simulink model "P2319ASW01"  (R2022b)
settings: configuration reference "SharedConfig" (kept outside this file)
libraries: simulink x3
settings Model: DataDictionary=P2319ASW01.sldd  Creator=Kevin  LastModifiedBy=Max Kolesnikov
settings ConfigSetRef: SourceName=SharedConfig

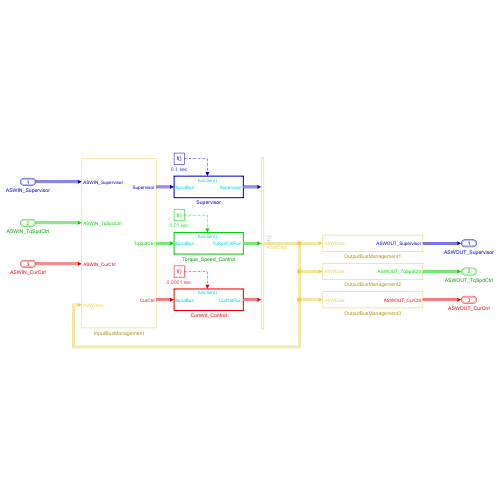
[thumbnail: Simulink's stored preview of the top-level diagram]
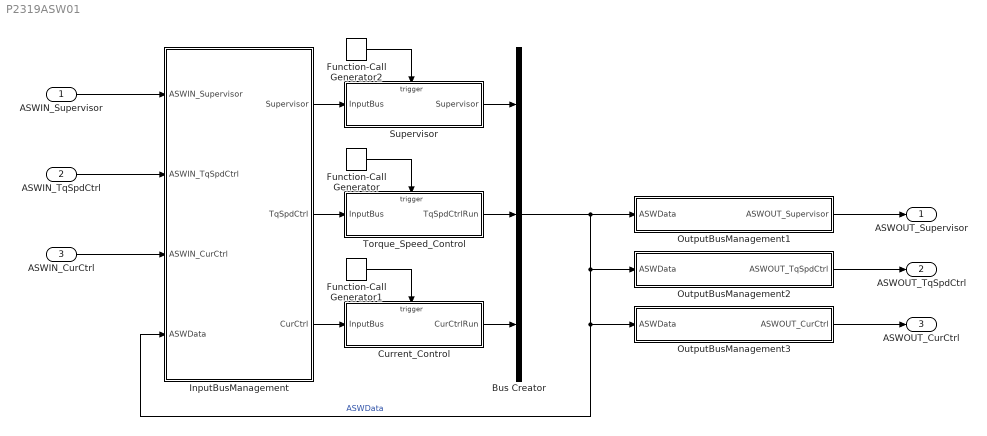
== system P2319ASW01 ==
  ASWIN_Supervisor : Inport  OutDataTypeStr=Bus: ASWIN_Supervisor
  ASWIN_TqSpdCtrl : Inport  Port=2  OutDataTypeStr=Bus: ASWIN_TqSpdCtrl
  ASWIN_CurCtrl : Inport  Port=3  OutDataTypeStr=Bus: ASWIN_CurCtrl
  Bus Creator : BusCreator  Inputs=3
  Current_Control : Subsystem  TreatAsAtomicUnit=on
      settings: RTWSystemCode=Nonreusable function
  Function-Call Generator : simulink/Ports & Subsystems/Function-Call Generator  sample_time=0.01  numberOfIterations=1  DisallowWideOutput=off
      settings: AttributesFormatString=%<sample_time> sec
  Function-Call Generator1 : simulink/Ports & Subsystems/Function-Call Generator  sample_time=0.0001  numberOfIterations=1  DisallowWideOutput=off
      settings: AttributesFormatString=%<sample_time> sec
  Function-Call Generator2 : simulink/Ports & Subsystems/Function-Call Generator  sample_time=0.1  numberOfIterations=1  DisallowWideOutput=off
      settings: AttributesFormatString=%<sample_time> sec
  InputBusManagement : Subsystem
  OutputBusManagement1 : Subsystem
  OutputBusManagement2 : Subsystem
  OutputBusManagement3 : Subsystem
  Supervisor : Subsystem  TreatAsAtomicUnit=on
      settings: RTWSystemCode=Nonreusable function
  Torque_Speed_Control : Subsystem  TreatAsAtomicUnit=on
      settings: RTWSystemCode=Nonreusable function
  ASWOUT_Supervisor : Outport  OutDataTypeStr=Bus: ASWOUT_Supervisor
  ASWOUT_TqSpdCtrl : Outport  Port=2  OutDataTypeStr=Bus: ASWOUT_TqSpdCtrl
  ASWOUT_CurCtrl : Outport  Port=3  OutDataTypeStr=Bus: ASWOUT_CurCtrl
  wires:
  Function-Call Generator/1 -> Torque_Speed_Control/Trigger
  Function-Call Generator2/1 -> Supervisor/Trigger
  Torque_Speed_Control/1(TqSpdCtrlRun) -> Bus Creator/2
  Supervisor/1(Supervisor) -> Bus Creator/1
  Current_Control/1(CurCtrlRun) -> Bus Creator/3
  Function-Call Generator1/1 -> Current_Control/Trigger
  Bus Creator/1 -> InputBusManagement/4(ASWData), OutputBusManagement3/1(ASWData), OutputBusManagement2/1(ASWData), OutputBusManagement1/1(ASWData)  "ASWData"
  InputBusManagement/1(Supervisor) -> Supervisor/1(InputBus)
  InputBusManagement/2(TqSpdCtrl) -> Torque_Speed_Control/1(InputBus)
  InputBusManagement/3(CurCtrl) -> Current_Control/1(InputBus)
  ASWIN_CurCtrl/1 -> InputBusManagement/3(ASWIN_CurCtrl)
  OutputBusManagement3/1(ASWOUT_CurCtrl) -> ASWOUT_CurCtrl/1
  OutputBusManagement1/1(ASWOUT_Supervisor) -> ASWOUT_Supervisor/1
  ASWIN_Supervisor/1 -> InputBusManagement/1(ASWIN_Supervisor)
  ASWIN_TqSpdCtrl/1 -> InputBusManagement/2(ASWIN_TqSpdCtrl)
  OutputBusManagement2/1(ASWOUT_TqSpdCtrl) -> ASWOUT_TqSpdCtrl/1

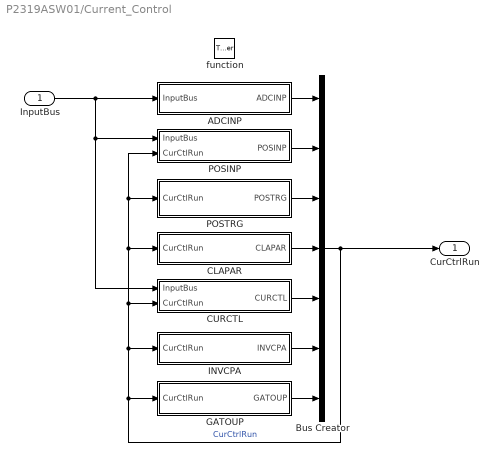
== system P2319ASW01/Current_Control ==
  InputBus : Inport
  function : TriggerPort  TriggerType=function-call  VariantControl=(inherit)
  ADCINP : Subsystem
  Bus Creator : BusCreator  Inputs=7
  CLAPAR : Subsystem
  CURCTL : Subsystem
  GATOUP : Subsystem
  INVCPA : Subsystem
  POSINP : Subsystem
  POSTRG : Subsystem
  CurCtrlRun : Outport
  wires:
  Bus Creator/1 -> CurCtrlRun/1, POSINP/2(CurCtlRun), POSTRG/1(CurCtlRun), CLAPAR/1(CurCtlRun), CURCTL/2(CurCtlRun), INVCPA/1(CurCtlRun), GATOUP/1(CurCtlRun)  "CurCtrlRun"
  POSINP/1(POSINP) -> Bus Creator/2
  ADCINP/1(ADCINP) -> Bus Creator/1
  POSTRG/1(POSTRG) -> Bus Creator/3
  CLAPAR/1(CLAPAR) -> Bus Creator/4
  CURCTL/1(CURCTL) -> Bus Creator/5
  INVCPA/1(INVCPA) -> Bus Creator/6
  GATOUP/1(GATOUP) -> Bus Creator/7
  InputBus/1 -> CURCTL/1(InputBus), POSINP/1(InputBus), ADCINP/1(InputBus)

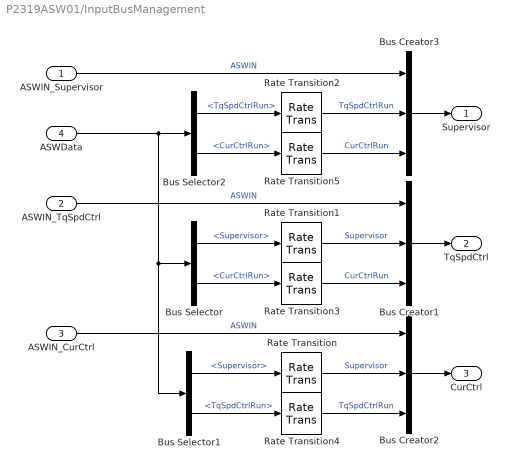
== system P2319ASW01/InputBusManagement ==
  ASWIN_Supervisor : Inport
  ASWIN_TqSpdCtrl : Inport  Port=2
  ASWIN_CurCtrl : Inport  Port=3
  ASWData : Inport  Port=4
  Bus Creator1 : BusCreator  Inputs=3
  Bus Creator2 : BusCreator  Inputs=3
  Bus Creator3 : BusCreator  Inputs=3
  Bus Selector : BusSelector  OutputSignals=Supervisor,CurCtrlRun
  Bus Selector1 : BusSelector  OutputSignals=Supervisor,TqSpdCtrlRun
  Bus Selector2 : BusSelector  OutputSignals=TqSpdCtrlRun,CurCtrlRun
  Rate Transition{,1..5} (6 alike) : RateTransition
  Supervisor : Outport
  TqSpdCtrl : Outport  Port=2
  CurCtrl : Outport  Port=3
  wires:
  Bus Selector1/1 -> Rate Transition/1  "<Supervisor>"
  Rate Transition3/1 -> Bus Creator1/3  "CurCtrlRun"
  Rate Transition4/1 -> Bus Creator2/3  "TqSpdCtrlRun"
  ASWIN_Supervisor/1 -> Bus Creator3/1  "ASWIN"
  Bus Selector/2 -> Rate Transition3/1  "<CurCtrlRun>"
  Bus Selector/1 -> Rate Transition1/1  "<Supervisor>"
  Rate Transition1/1 -> Bus Creator1/2  "Supervisor"
  Bus Selector1/2 -> Rate Transition4/1  "<TqSpdCtrlRun>"
  Rate Transition/1 -> Bus Creator2/2  "Supervisor"
  Bus Creator2/1 -> CurCtrl/1
  Bus Creator1/1 -> TqSpdCtrl/1
  ASWIN_CurCtrl/1 -> Bus Creator2/1  "ASWIN"
  ASWIN_TqSpdCtrl/1 -> Bus Creator1/1  "ASWIN"
  Bus Creator3/1 -> Supervisor/1
  Rate Transition2/1 -> Bus Creator3/2  "TqSpdCtrlRun"
  Bus Selector2/1 -> Rate Transition2/1  "<TqSpdCtrlRun>"
  Bus Selector2/2 -> Rate Transition5/1  "<CurCtrlRun>"
  Rate Transition5/1 -> Bus Creator3/3  "CurCtrlRun"
  ASWData/1 -> Bus Selector1/1, Bus Selector/1, Bus Selector2/1

== system P2319ASW01/OutputBusManagement1 ==
  ASWData : Inport
  Bus Creator : BusCreator  Inputs=10
  Bus Selector : BusSelector  OutputSignals=Supervisor.SLWOUP.ASWOUT_GreenLed,Supervisor.SLWOUP.ASWOUT_RedLed,Supervisor.SLWOUP.ASWOUT_YellowLed,Supervisor.SLWOUP.ASWOUT_ResolverExctEna,Supervisor.SLWOUP.ASWOUT_McuData2Da,Supervisor.SLWOUP.ASWOUT_CanPwrPwmEna,Supervisor.SLWOUP.ASWOUT_InPwrPwmEna,Supervisor.SLWOUP.ASWOUT_MtrPwrPwmEna,Supervisor.SLWOUP.ASWOUT_SwPwrPwmEna,Supervisor.SLWOUP.ASWOUT_PhaPwmEna
  ASWOUT_Supervisor : Outport
  wires:
  Bus Creator/1 -> ASWOUT_Supervisor/1
  ASWData/1 -> Bus Selector/1
  Bus Selector/1 -> Bus Creator/1  "<ASWOUT_GreenLed>"
  Bus Selector/2 -> Bus Creator/2  "<ASWOUT_RedLed>"
  Bus Selector/3 -> Bus Creator/3  "<ASWOUT_YellowLed>"
  Bus Selector/4 -> Bus Creator/4  "<ASWOUT_ResolverExctEna>"
  Bus Selector/5 -> Bus Creator/5  "<ASWOUT_McuData2Da>"
  Bus Selector/6 -> Bus Creator/6  "<ASWOUT_CanPwrPwmEna>"
  Bus Selector/9 -> Bus Creator/9  "<ASWOUT_SwPwrPwmEna>"
  Bus Selector/8 -> Bus Creator/8  "<ASWOUT_MtrPwrPwmEna>"
  Bus Selector/10 -> Bus Creator/10  "<ASWOUT_PhaPwmEna>"
  Bus Selector/7 -> Bus Creator/7  "<ASWOUT_InPwrPwmEna>"

== system P2319ASW01/OutputBusManagement2 ==
  ASWData : Inport
  Bus Creator : BusCreator  Inputs=1
  Bus Selector : BusSelector  OutputSignals=TqSpdCtrlRun.MEDOUP.ASWOUT_McuData1Da
  ASWOUT_TqSpdCtrl : Outport
  wires:
  ASWData/1 -> Bus Selector/1
  Bus Creator/1 -> ASWOUT_TqSpdCtrl/1
  Bus Selector/1 -> Bus Creator/1  "<ASWOUT_McuData1Da>"

== system P2319ASW01/OutputBusManagement3 ==
  ASWData : Inport
  Bus Creator : BusCreator  Inputs=3
  Bus Selector : BusSelector  OutputSignals=CurCtrlRun.GATOUP.ASWOUT_PhaAPwmDc,CurCtrlRun.GATOUP.ASWOUT_PhaBPwmDc,CurCtrlRun.GATOUP.ASWOUT_PhaCPwmDc
  ASWOUT_CurCtrl : Outport
  wires:
  ASWData/1 -> Bus Selector/1
  Bus Creator/1 -> ASWOUT_CurCtrl/1
  Bus Selector/1 -> Bus Creator/1  "<ASWOUT_PhaAPwmDc>"
  Bus Selector/2 -> Bus Creator/2  "<ASWOUT_PhaBPwmDc>"
  Bus Selector/3 -> Bus Creator/3  "<ASWOUT_PhaCPwmDc>"

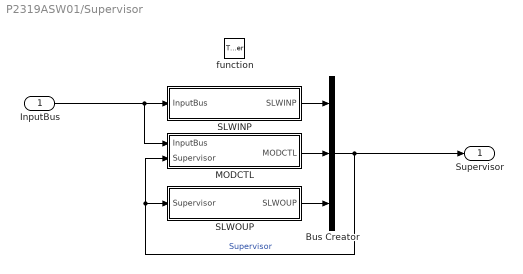
== system P2319ASW01/Supervisor ==
  InputBus : Inport
  function : TriggerPort  TriggerType=function-call  VariantControl=(inherit)
  Bus Creator : BusCreator  Inputs=3
  MODCTL : Subsystem
  SLWINP : Subsystem
  SLWOUP : Subsystem
  Supervisor : Outport
  wires:
  Bus Creator/1 -> Supervisor/1, SLWOUP/1(Supervisor), MODCTL/2(Supervisor)  "Supervisor"
  MODCTL/1(MODCTL) -> Bus Creator/2
  SLWINP/1(SLWINP) -> Bus Creator/1
  SLWOUP/1(SLWOUP) -> Bus Creator/3
  InputBus/1 -> MODCTL/1(InputBus), SLWINP/1(InputBus)

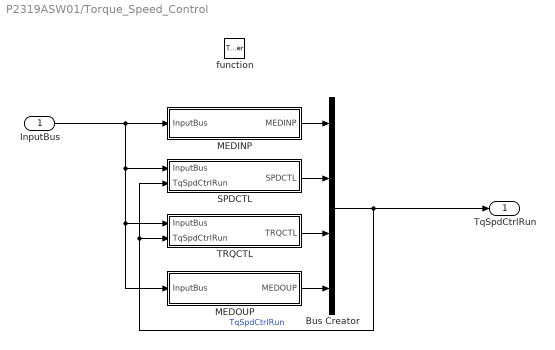
== system P2319ASW01/Torque_Speed_Control ==
  InputBus : Inport
  function : TriggerPort  TriggerType=function-call  VariantControl=(inherit)
  Bus Creator : BusCreator  Inputs=4
  MEDINP : Subsystem
  MEDOUP : Subsystem
  SPDCTL : Subsystem
  TRQCTL : Subsystem
  TqSpdCtrlRun : Outport
  wires:
  Bus Creator/1 -> TqSpdCtrlRun/1, SPDCTL/2(TqSpdCtrlRun), TRQCTL/2(TqSpdCtrlRun)  "TqSpdCtrlRun"
  SPDCTL/1(SPDCTL) -> Bus Creator/2
  TRQCTL/1(TRQCTL) -> Bus Creator/3
  MEDINP/1(MEDINP) -> Bus Creator/1
  MEDOUP/1(MEDOUP) -> Bus Creator/4
  InputBus/1 -> MEDINP/1(InputBus), MEDOUP/1(InputBus), TRQCTL/1(InputBus), SPDCTL/1(InputBus)

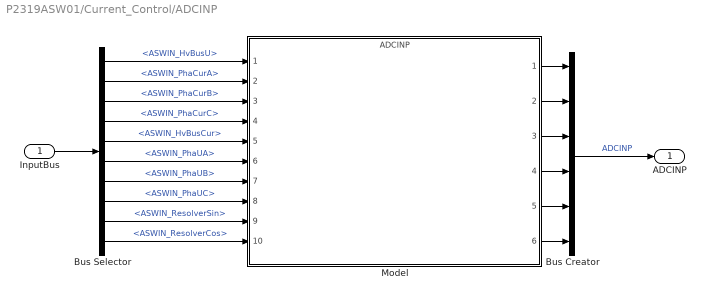
== system P2319ASW01/Current_Control/ADCINP ==
  InputBus : Inport
  Bus Creator : BusCreator  Inputs=6
  Bus Selector : BusSelector  OutputSignals=ASWIN.ASWIN_HvBusU,ASWIN.ASWIN_PhaCurA,ASWIN.ASWIN_PhaCurB,ASWIN.ASWIN_PhaCurC,ASWIN.ASWIN_HvBusCur,ASWIN.ASWIN_PhaUA,ASWIN.ASWIN_PhaUB,ASWIN.ASWIN_PhaUC,ASWIN.ASWIN_ResolverSin,ASWIN.ASWIN_ResolverCos
  Model : ModelReference  ModelNameDialog=ADCINP.slx  SimulationMode=Normal  ModelReferenceVersion=1.80
  ADCINP : Outport
  wires:
  Model/1 -> Bus Creator/1
  Model/2 -> Bus Creator/2
  Bus Creator/1 -> ADCINP/1  "ADCINP"
  Model/3 -> Bus Creator/3
  Model/4 -> Bus Creator/4
  InputBus/1 -> Bus Selector/1
  Model/5 -> Bus Creator/5
  Bus Selector/1 -> Model/1  "<ASWIN_HvBusU>"
  Bus Selector/2 -> Model/2  "<ASWIN_PhaCurA>"
  Bus Selector/3 -> Model/3  "<ASWIN_PhaCurB>"
  Bus Selector/4 -> Model/4  "<ASWIN_PhaCurC>"
  Bus Selector/5 -> Model/5  "<ASWIN_HvBusCur>"
  Bus Selector/6 -> Model/6  "<ASWIN_PhaUA>"
  Bus Selector/7 -> Model/7  "<ASWIN_PhaUB>"
  Bus Selector/8 -> Model/8  "<ASWIN_PhaUC>"
  Bus Selector/9 -> Model/9  "<ASWIN_ResolverSin>"
  Bus Selector/10 -> Model/10  "<ASWIN_ResolverCos>"
  Model/6 -> Bus Creator/6

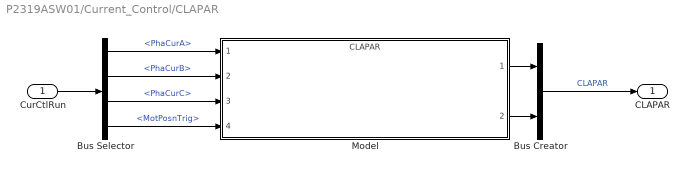
== system P2319ASW01/Current_Control/CLAPAR ==
  CurCtlRun : Inport
  Bus Creator : BusCreator  Inputs=2
  Bus Selector : BusSelector  OutputSignals=ADCINP.PhaCurA,ADCINP.PhaCurB,ADCINP.PhaCurC,POSTRG.MotPosnTrig
  Model : ModelReference  ModelNameDialog=CLAPAR.slx  SimulationMode=Normal  ModelReferenceVersion=1.48
  CLAPAR : Outport
  wires:
  CurCtlRun/1 -> Bus Selector/1
  Model/1 -> Bus Creator/1
  Model/2 -> Bus Creator/2
  Bus Creator/1 -> CLAPAR/1  "CLAPAR"
  Bus Selector/4 -> Model/4  "<MotPosnTrig>"
  Bus Selector/3 -> Model/3  "<PhaCurC>"
  Bus Selector/2 -> Model/2  "<PhaCurB>"
  Bus Selector/1 -> Model/1  "<PhaCurA>"

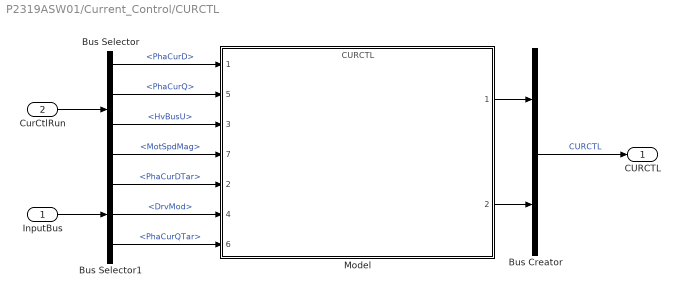
== system P2319ASW01/Current_Control/CURCTL ==
  InputBus : Inport
  CurCtlRun : Inport  Port=2
  Bus Creator : BusCreator  Inputs=2
  Bus Selector : BusSelector  OutputSignals=CLAPAR.PhaCurD,CLAPAR.PhaCurQ,ADCINP.HvBusU,POSINP.MotSpdMag
  Bus Selector1 : BusSelector  OutputSignals=TqSpdCtrlRun.TRQCTL.PhaCurDTar,Supervisor.MODCTL.DrvMod,TqSpdCtrlRun.TRQCTL.PhaCurQTar
  Model : ModelReference  ModelNameDialog=CURCTL.slx  SimulationMode=Normal  ModelReferenceVersion=1.185
      settings: PortSchema="{\"entries\":[{\"content\":{\"sides\":[{\"content\":{\"connectorIds\":[\"In1\",\"In5\",\"In3\",\"In7\",\"In2\",\"In4\",\"In6\"]},\"type\":\"ConnectorPlacement.EquallySpacedRectSide\",\"uuid\":\"db0f62ab-31b9-42f9-9795-c2675c3253e4\"},{\"content\":{\"connectorIds\":[\"Out1\",\"Out2\"],\"side\":\"RIGHT\"},\"type\":\"ConnectorPlacement.EquallySpacedRectSide\",\"uuid\":\"434672ae-ba7a-456a-995b-f16636dd9977\"},{\"content\":{\"connectorIds\":[],\"side\":\"TOP\"},\"type\":\"ConnectorPlacement.EquallySpacedRectSide\",\"uuid\":\"d643b050-5ed5-4272-be3e-445ed132b13e\"}]},\"type\":\"ConnectorPlacement.EquallySpacedConnector\",\"uuid\":\"f814aeaf-6b06-4bbb-9974-79572176904c\"}],\"packageUris\":[\"http://schema.mathworks.com/mf0/Connector/R2020b\"],\"version\":\"1.0\"}"
  CURCTL : Outport
  wires:
  Bus Creator/1 -> CURCTL/1  "CURCTL"
  Model/2 -> Bus Creator/2
  Model/1 -> Bus Creator/1
  CurCtlRun/1 -> Bus Selector/1
  Bus Selector/1 -> Model/1  "<PhaCurD>"
  Bus Selector/2 -> Model/5  "<PhaCurQ>"
  InputBus/1 -> Bus Selector1/1
  Bus Selector1/1 -> Model/2  "<PhaCurDTar>"
  Bus Selector1/2 -> Model/4  "<DrvMod>"
  Bus Selector1/3 -> Model/6  "<PhaCurQTar>"
  Bus Selector/3 -> Model/3  "<HvBusU>"
  Bus Selector/4 -> Model/7  "<MotSpdMag>"

== system P2319ASW01/Current_Control/GATOUP ==
  CurCtlRun : Inport
  Bus Creator : BusCreator  Inputs=3
  Bus Selector : BusSelector  OutputSignals=INVCPA.PhaUACmd,INVCPA.PhaUBCmd,INVCPA.PhaUCCmd,ADCINP.HvBusU
  Model : ModelReference  ModelNameDialog=GATOUP.slx  SimulationMode=Normal  ModelReferenceVersion=1.75
  GATOUP : Outport
  wires:
  Bus Selector/3 -> Model/3  "<PhaUCCmd>"
  Bus Selector/2 -> Model/2  "<PhaUBCmd>"
  Bus Selector/1 -> Model/1  "<PhaUACmd>"
  Model/3 -> Bus Creator/3
  Model/2 -> Bus Creator/2
  Model/1 -> Bus Creator/1
  Bus Creator/1 -> GATOUP/1  "GATOUP"
  CurCtlRun/1 -> Bus Selector/1
  Bus Selector/4 -> Model/4  "<HvBusU>"

== system P2319ASW01/Current_Control/INVCPA ==
  CurCtlRun : Inport
  Bus Creator : BusCreator  Inputs=3
  Bus Selector : BusSelector  OutputSignals=CURCTL.PhaUDCmd,CURCTL.PhaUQCmd,POSTRG.MotPosnTrig
  Model : ModelReference  ModelNameDialog=INVCPA.slx  SimulationMode=Normal  ModelReferenceVersion=1.40
  INVCPA : Outport
  wires:
  CurCtlRun/1 -> Bus Selector/1
  Bus Creator/1 -> INVCPA/1  "INVCPA"
  Model/1 -> Bus Creator/1
  Model/2 -> Bus Creator/2
  Model/3 -> Bus Creator/3
  Bus Selector/1 -> Model/1  "<PhaUDCmd>"
  Bus Selector/2 -> Model/2  "<PhaUQCmd>"
  Bus Selector/3 -> Model/3  "<MotPosnTrig>"

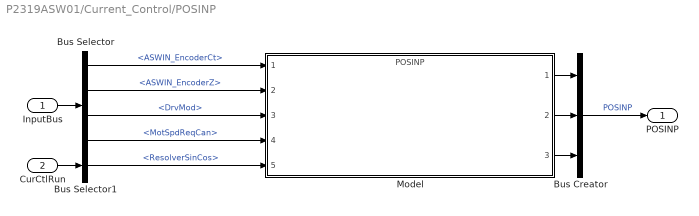
== system P2319ASW01/Current_Control/POSINP ==
  InputBus : Inport
  CurCtlRun : Inport  Port=2
  Bus Creator : BusCreator  Inputs=3
  Bus Selector : BusSelector  OutputSignals=ASWIN.ASWIN_EncoderCt,ASWIN.ASWIN_EncoderZ,Supervisor.MODCTL.DrvMod,TqSpdCtrlRun.MEDINP.MotSpdReqCan
  Bus Selector1 : BusSelector  OutputSignals=ADCINP.ResolverSinCos
  Model : ModelReference  ModelNameDialog=POSINP.slx  SimulationMode=Normal  ModelReferenceVersion=1.188
  POSINP : Outport
  wires:
  Bus Creator/1 -> POSINP/1  "POSINP"
  InputBus/1 -> Bus Selector/1
  Model/1 -> Bus Creator/1
  Bus Selector/2 -> Model/2  "<ASWIN_EncoderZ>"
  Bus Selector/1 -> Model/1  "<ASWIN_EncoderCt>"
  Model/2 -> Bus Creator/2
  Bus Selector/3 -> Model/3  "<DrvMod>"
  Bus Selector/4 -> Model/4  "<MotSpdReqCan>"
  Model/3 -> Bus Creator/3
  CurCtlRun/1 -> Bus Selector1/1
  Bus Selector1/1 -> Model/5  "<ResolverSinCos>"

== system P2319ASW01/Current_Control/POSTRG ==
  CurCtlRun : Inport
  Bus Creator : BusCreator  Inputs=1
  Bus Selector : BusSelector  OutputSignals=POSINP.MotPosnMag
  Model : ModelReference  ModelNameDialog=POSTRG.slx  SimulationMode=Normal  ModelReferenceVersion=1.184
  POSTRG : Outport
  wires:
  Bus Creator/1 -> POSTRG/1  "POSTRG"
  CurCtlRun/1 -> Bus Selector/1
  Bus Selector/1 -> Model/1  "<MotPosnMag>"
  Model/1 -> Bus Creator/1

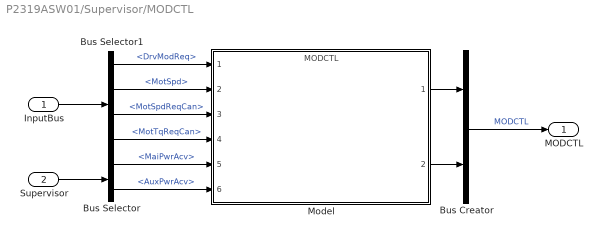
== system P2319ASW01/Supervisor/MODCTL ==
  InputBus : Inport
  Supervisor : Inport  Port=2
  Bus Creator : BusCreator  Inputs=2
  Bus Selector : BusSelector  OutputSignals=SLWINP.MaiPwrAcv,SLWINP.AuxPwrAcv
  Bus Selector1 : BusSelector  OutputSignals=TqSpdCtrlRun.MEDINP.DrvModReq,CurCtrlRun.POSINP.MotSpd,TqSpdCtrlRun.MEDINP.MotSpdReqCan,TqSpdCtrlRun.MEDINP.MotTqReqCan
  Model : ModelReference  ModelNameDialog=MODCTL.slx  SimulationMode=Normal  ModelReferenceVersion=1.60
  MODCTL : Outport
  wires:
  Bus Creator/1 -> MODCTL/1  "MODCTL"
  Model/1 -> Bus Creator/1
  Supervisor/1 -> Bus Selector/1
  Model/2 -> Bus Creator/2
  Bus Selector/2 -> Model/6  "<AuxPwrAcv>"
  Bus Selector/1 -> Model/5  "<MaiPwrAcv>"
  InputBus/1 -> Bus Selector1/1
  Bus Selector1/2 -> Model/2  "<MotSpd>"
  Bus Selector1/1 -> Model/1  "<DrvModReq>"
  Bus Selector1/3 -> Model/3  "<MotSpdReqCan>"
  Bus Selector1/4 -> Model/4  "<MotTqReqCan>"

== system P2319ASW01/Supervisor/SLWINP ==
  InputBus : Inport
  Bus Creator : BusCreator  Inputs=5
  Bus Selector : BusSelector  OutputSignals=ASWIN.ASWIN_MaiPwrSts,ASWIN.ASWIN_AuxPwrSts,ASWIN.ASWIN_BdT1,ASWIN.ASWIN_BdT2,ASWIN.ASWIN_McuURef,ASWIN.ASWIN_McuT,ASWIN.ASWIN_McuUBat
  Model : ModelReference  ModelNameDialog=SLWINP.slx  SimulationMode=Normal  ModelReferenceVersion=1.60
  SLWINP : Outport
  wires:
  InputBus/1 -> Bus Selector/1
  Model/1 -> Bus Creator/1
  Bus Creator/1 -> SLWINP/1  "SLWINP"
  Model/2 -> Bus Creator/2
  Model/3 -> Bus Creator/3
  Model/4 -> Bus Creator/4
  Model/5 -> Bus Creator/5
  Bus Selector/1 -> Model/1  "<ASWIN_MaiPwrSts>"
  Bus Selector/2 -> Model/2  "<ASWIN_AuxPwrSts>"
  Bus Selector/3 -> Model/3  "<ASWIN_BdT1>"
  Bus Selector/4 -> Model/4  "<ASWIN_BdT2>"
  Bus Selector/5 -> Model/5  "<ASWIN_McuURef>"
  Bus Selector/6 -> Model/6  "<ASWIN_McuT>"
  Bus Selector/7 -> Model/7  "<ASWIN_McuUBat>"

== system P2319ASW01/Supervisor/SLWOUP ==
  Supervisor : Inport
  Bus Creator : BusCreator  Inputs=10
  Bus Selector : BusSelector  OutputSignals=MODCTL.DrvMod,MODCTL.PwrCmd,SLWINP.BdT1,SLWINP.BdT2,SLWINP.McuT
  Model : ModelReference  ModelNameDialog=SLWOUP.slx  SimulationMode=Normal  ModelReferenceVersion=1.65
  SLWOUP : Outport
  wires:
  Model/5 -> Bus Creator/5
  Model/4 -> Bus Creator/4
  Model/3 -> Bus Creator/3
  Model/2 -> Bus Creator/2
  Bus Creator/1 -> SLWOUP/1  "SLWOUP"
  Model/1 -> Bus Creator/1
  Supervisor/1 -> Bus Selector/1
  Bus Selector/1 -> Model/1  "<DrvMod>"
  Bus Selector/2 -> Model/2  "<PwrCmd>"
  Bus Selector/3 -> Model/3  "<BdT1>"
  Bus Selector/4 -> Model/4  "<BdT2>"
  Bus Selector/5 -> Model/5  "<McuT>"
  Model/6 -> Bus Creator/6
  Model/7 -> Bus Creator/7
  Model/8 -> Bus Creator/8
  Model/9 -> Bus Creator/9
  Model/10 -> Bus Creator/10

== system P2319ASW01/Torque_Speed_Control/MEDINP ==
  InputBus : Inport
  Bus Creator : BusCreator  Inputs=3
  Bus Selector : BusSelector  OutputSignals=ASWIN.ASWIN_McuReqDa,ASWIN.ASWIN_McuReqCt
  Model : ModelReference  ModelNameDialog=MEDINP.slx  SimulationMode=Normal  ModelReferenceVersion=1.36
  MEDINP : Outport
  wires:
  Model/1 -> Bus Creator/1
  InputBus/1 -> Bus Selector/1
  Bus Creator/1 -> MEDINP/1  "MEDINP"
  Model/2 -> Bus Creator/2
  Model/3 -> Bus Creator/3
  Bus Selector/1 -> Model/1  "<ASWIN_McuReqDa>"
  Bus Selector/2 -> Model/2  "<ASWIN_McuReqCt>"

== system P2319ASW01/Torque_Speed_Control/MEDOUP ==
  InputBus : Inport
  Bus Creator : BusCreator  Inputs=1
  Bus Selector : BusSelector  OutputSignals=CurCtrlRun.ADCINP.HvBusCur,CurCtrlRun.ADCINP.HvBusU,CurCtrlRun.CLAPAR.PhaCurQ,CurCtrlRun.POSINP.MotSpd,Supervisor.MODCTL.DrvMod
  Model : ModelReference  ModelNameDialog=MEDOUP.slx  SimulationMode=Normal  ModelReferenceVersion=1.21
  MEDOUP : Outport
  wires:
  Bus Creator/1 -> MEDOUP/1  "MEDOUP"
  Model/1 -> Bus Creator/1
  InputBus/1 -> Bus Selector/1
  Bus Selector/3 -> Model/3  "<PhaCurQ>"
  Bus Selector/4 -> Model/4  "<MotSpd>"
  Bus Selector/2 -> Model/2  "<HvBusU>"
  Bus Selector/5 -> Model/5  "<DrvMod>"
  Bus Selector/1 -> Model/1  "<HvBusCur>"

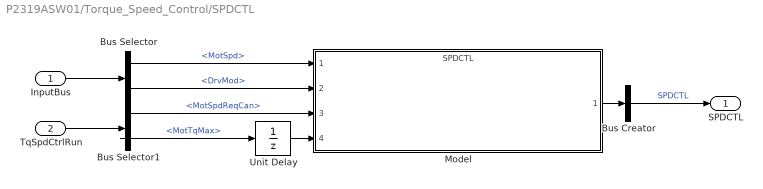
== system P2319ASW01/Torque_Speed_Control/SPDCTL ==
  InputBus : Inport
  TqSpdCtrlRun : Inport  Port=2
  Bus Creator : BusCreator  Inputs=1
  Bus Selector : BusSelector  OutputSignals=CurCtrlRun.POSINP.MotSpd,Supervisor.MODCTL.DrvMod
  Bus Selector1 : BusSelector  OutputSignals=MEDINP.MotSpdReqCan,TRQCTL.MotTqMax
  Model : ModelReference  ModelNameDialog=SPDCTL.slx  SimulationMode=Normal  ModelReferenceVersion=1.79
  Unit Delay : UnitDelay  SampleTime=-1  HasFrameUpgradeWarning=on
  SPDCTL : Outport
  wires:
  Bus Creator/1 -> SPDCTL/1  "SPDCTL"
  InputBus/1 -> Bus Selector/1
  Model/1 -> Bus Creator/1
  Bus Selector/2 -> Model/2  "<DrvMod>"
  Bus Selector/1 -> Model/1  "<MotSpd>"
  TqSpdCtrlRun/1 -> Bus Selector1/1
  Bus Selector1/1 -> Model/3  "<MotSpdReqCan>"
  Bus Selector1/2 -> Unit Delay/1  "<MotTqMax>"
  Unit Delay/1 -> Model/4

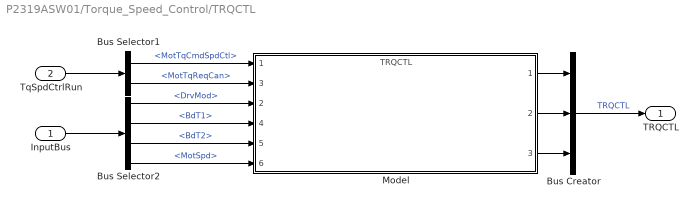
== system P2319ASW01/Torque_Speed_Control/TRQCTL ==
  InputBus : Inport
  TqSpdCtrlRun : Inport  Port=2
  Bus Creator : BusCreator  Inputs=3
  Bus Selector1 : BusSelector  OutputSignals=SPDCTL.MotTqCmdSpdCtl,MEDINP.MotTqReqCan
  Bus Selector2 : BusSelector  OutputSignals=Supervisor.MODCTL.DrvMod,Supervisor.SLWINP.BdT1,Supervisor.SLWINP.BdT2,CurCtrlRun.POSINP.MotSpd
  Model : ModelReference  ModelNameDialog=TRQCTL.slx  SimulationMode=Normal  ModelReferenceVersion=1.70
      settings: PortSchema="{\"entries\":[{\"content\":{\"sides\":[{\"content\":{\"connectorIds\":[\"In1\",\"In3\",\"In2\",\"In4\",\"In5\",\"In6\"]},\"type\":\"ConnectorPlacement.EquallySpacedRectSide\",\"uuid\":\"a2036680-d12c-48a4-a5d4-964115010c8b\"},{\"content\":{\"connectorIds\":[\"Out1\",\"Out2\",\"Out3\"],\"side\":\"RIGHT\"},\"type\":\"ConnectorPlacement.EquallySpacedRectSide\",\"uuid\":\"d029f408-d507-4823-8c0e-ee4992dac706\"},{\"content\":{\"connectorIds\":[],\"side\":\"TOP\"},\"type\":\"ConnectorPlacement.EquallySpacedRectSide\",\"uuid\":\"76cfb08c-b345-4a08-913a-65da3c0086d2\"}]},\"type\":\"ConnectorPlacement.EquallySpacedConnector\",\"uuid\":\"1b06f88e-2083-42a2-9621-3b42e52dcd4a\"}],\"packageUris\":[\"http://schema.mathworks.com/mf0/Connector/R2020b\"],\"version\":\"1.0\"}"
  TRQCTL : Outport
  wires:
  Model/1 -> Bus Creator/1
  InputBus/1 -> Bus Selector2/1
  Bus Creator/1 -> TRQCTL/1  "TRQCTL"
  Model/2 -> Bus Creator/2
  TqSpdCtrlRun/1 -> Bus Selector1/1
  Bus Selector1/1 -> Model/1  "<MotTqCmdSpdCtl>"
  Bus Selector1/2 -> Model/3  "<MotTqReqCan>"
  Bus Selector2/1 -> Model/2  "<DrvMod>"
  Model/3 -> Bus Creator/3
  Bus Selector2/2 -> Model/4  "<BdT1>"
  Bus Selector2/3 -> Model/5  "<BdT2>"
  Bus Selector2/4 -> Model/6  "<MotSpd>"
